simulink model "Hinf_scheme"  (R2019b)
settings: Solver=VariableStepAuto  StartTime=0.0  StopTime=10.0  RelTol=1e-3
values from neighbouring files (symbols this model uses):
  data = e_h.load_data    [potentiometer_recover.m]
  experiment = merge( experiment, experiment2 )    [blackbox_est.m]
libraries: simulink x5, cstblocks x3
settings Model: Creator=giacomo  LastModifiedBy=giacomo

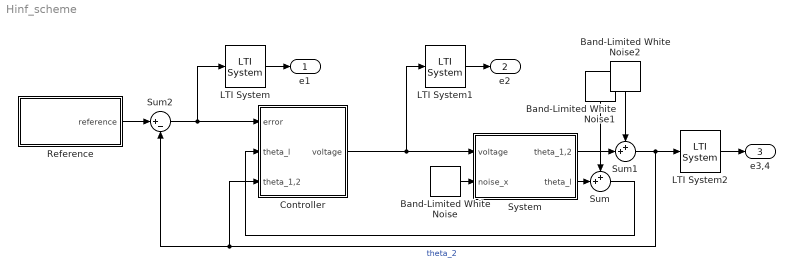
== system Hinf_scheme ==
  Band-Limited White Noise : simulink/Sources/Band-Limited White Noise  Cov=[0.1]  Ts=0.1  seed=[23341]
  Band-Limited White Noise1 : simulink/Sources/Band-Limited White Noise  Cov=[0.1]  Ts=0.1  seed=[23341]
  Band-Limited White Noise2 : simulink/Sources/Band-Limited White Noise  Cov=[0.1]  Ts=0.1  seed=[23341]
  Controller : Subsystem
  LTI System : cstblocks/LTI System  sys=W_e  IC=[]
  LTI System1 : cstblocks/LTI System  sys=W_u  IC=[]
  LTI System2 : cstblocks/LTI System  sys=W_t12  IC=[]
  Reference : Subsystem
  Sum : Sum  Inputs=++|
  Sum1 : Sum  Inputs=++|
  Sum2 : Sum  Inputs=|+-
  System : Subsystem
  e1 : Outport
  e2 : Outport  Port=2
  e3,4 : Outport  Port=3
  wires:
  Sum/1 -> Controller/2(theta_l)
  Reference/1(reference) -> Sum2/1
  Sum2/1 -> LTI System/1, Controller/1(error)
  Controller/1(voltage) -> LTI System1/1, System/1(voltage)
  Band-Limited White Noise/1 -> System/2(noise_x)
  Sum1/1 -> Sum2/2, Controller/3(theta_1,2), LTI System2/1  "theta_2"
  System/1(theta_1,2) -> Sum1/2
  System/2(theta_l) -> Sum/2
  Band-Limited White Noise1/1 -> Sum/1
  Band-Limited White Noise2/1 -> Sum1/1
  LTI System/1 -> e1/1
  LTI System1/1 -> e2/1
  LTI System2/1 -> e3,4/1

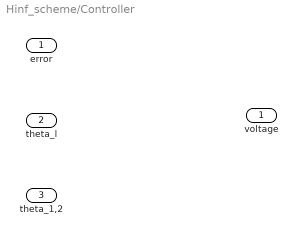
== system Hinf_scheme/Controller ==
  error : Inport
  theta_l : Inport  Port=2
  theta_1,2 : Inport  Port=3
  voltage : Outport

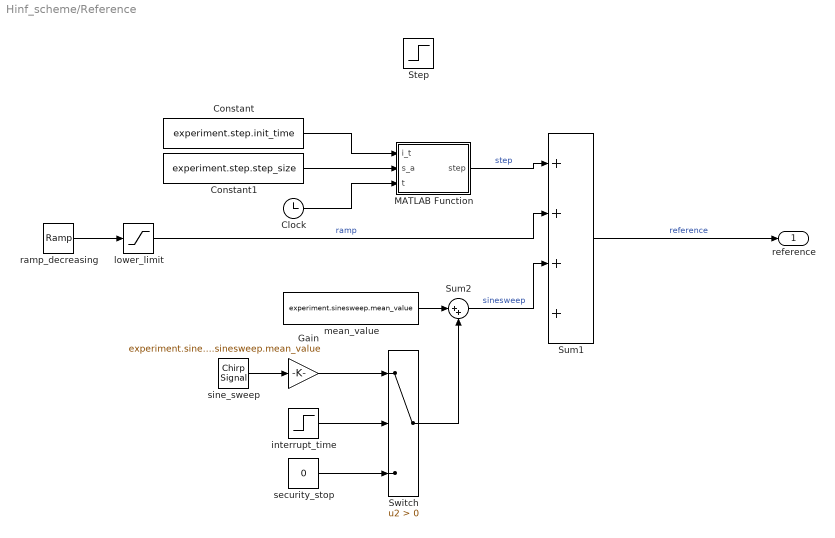
== system Hinf_scheme/Reference ==
  Clock : Clock
  Constant : Constant  Value=experiment.step.init_time
  Constant1 : Constant  Value=experiment.step.step_size
  Gain : Gain  Gain=experiment.sinesweep.v_max-experiment.sinesweep.mean_value
  MATLAB Function : MATLAB Function  TreatAsAtomicUnit=on
  Step : Step  Before=-data.motor_pos_0  After=0  SampleTime=0
  Sum1 : Sum  Inputs=++++
  Sum2 : Sum  Inputs=|++
  Switch : Switch  Criteria=u2 > Threshold
  interrupt_time : Step  Time=experiment.sinesweep.target_time  Before=1  After=-1  SampleTime=0
  lower_limit : Saturate  UpperLimit=max( experiment.ramp.init_value, experiment.ramp.final_value )  LowerLimit=min( experiment.ramp.init_value, experiment.ramp.final_value )
  mean_value : Constant  Value=experiment.sinesweep.mean_value
  ramp_decreasing : simulink/Sources/Ramp  slope=experiment.ramp.ramp_pend  start=experiment.ramp.init_time  InitialOutput=experiment.ramp.init_value
  security_stop : Constant  Value=0
  sine_sweep : simulink/Sources/Chirp Signal  f1=experiment.sinesweep.init_freq  T=experiment.sinesweep.target_time  f2=experiment.sinesweep.final_freq
  reference : Outport
  wires:
  mean_value/1 -> Sum2/1
  lower_limit/1 -> Sum1/2  "ramp"
  Switch/1 -> Sum2/2
  interrupt_time/1 -> Switch/2
  Sum2/1 -> Sum1/3  "sinesweep"
  Sum1/1 -> reference/1  "reference"
  security_stop/1 -> Switch/3
  ramp_decreasing/1 -> lower_limit/1
  Gain/1 -> Switch/1
  sine_sweep/1 -> Gain/1
  Clock/1 -> MATLAB Function/3(t)
  Constant/1 -> MATLAB Function/1(i_t)
  Constant1/1 -> MATLAB Function/2(s_a)
  MATLAB Function/1(step) -> Sum1/1  "step"

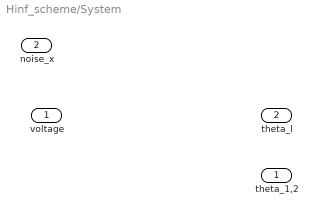
== system Hinf_scheme/System ==
  voltage : Inport
  noise_x : Inport  Port=2
  theta_1,2 : Outport
  theta_l : Outport  Port=2

== matlab function Hinf_scheme/Reference/MATLAB Function ==
  data: i_t input; step output; s_a input; t input
function step = multistep(i_t, s_a, t)

% it is assumed i_t is sorted!

% find the first time step that is greater than actual time. 
step = 0;
for idx = 1:length(i_t) 
    if i_t(idx) <= t
        step = s_a(idx);
    end
end
